simulink model "oppg5_5_e"  (R2015a)
settings: Solver=ode45  StartTime=0.0  StopTime=600  RelTol=1e-3
values from neighbouring files (symbols this model uses):
  K_pd = sqrt(T_f^2*omega_c^4+omega_c^2)/K    [oppg5_3_a.m]
  T = double(T)    [FindParam.m]    (also in oppg5_3_a.m)
  T_f = -1/(omega_c*tan(130*pi/180))    [oppg5_3_a.m]
libraries: simulink x2
settings Model: Creator=markh  LastModifiedBy=mikhailv
settings DataIOCC: SignalLoggingSaveFormat=ModelDataLogs  SignalLoggingName=sigsOut
settings OptimizationCC: InitFltsAndDblsToZero=on
settings DebuggingCC: SaveWithParameterizedLinksMsg=none  UnderspecifiedInitializationDetection=Classic  MergeDetectMultiDrivingBlocksExec=none  SignalResolutionControl=TryResolveAllWithWarning  MultiTaskDSMMsg=warning  MultiTaskCondExecSysMsg=none  FcnCallInpInsideContextMsg=UseLocalSettings  StateNameClashWarn=warning
settings HardwareCC: TargetUnknown=on
settings GRTTargetCC: TargetFcnLib=ansi_tfl_tmw.mat  CombineOutputUpdateFcns=off  GRTInterface=on

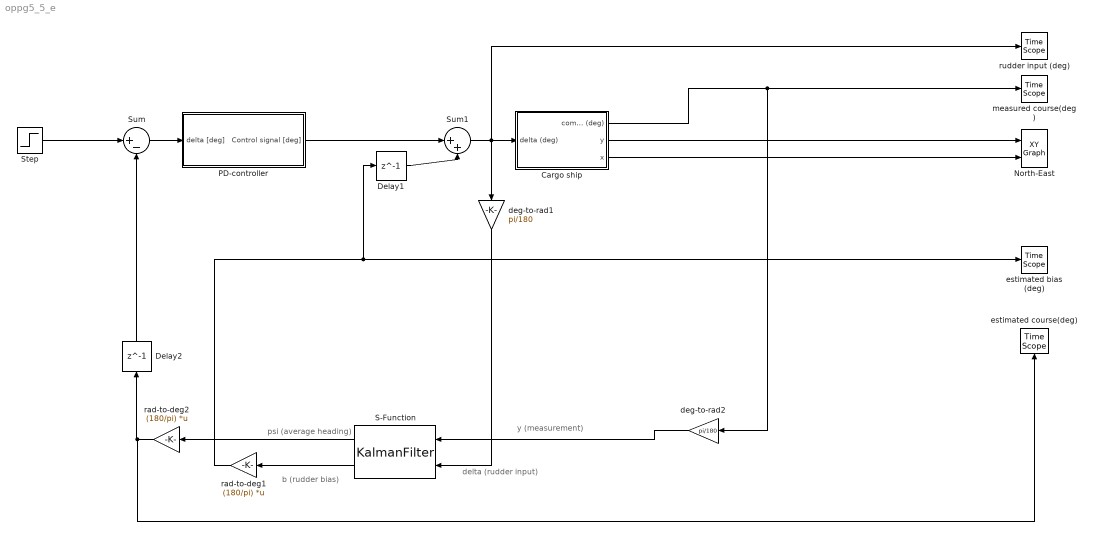
== system oppg5_5_e ==
  note: delta (rudder input)
  note: y (measurement)
  note: b (rudder bias)
  note: psi (average heading)
  Cargo ship : Subsystem  mask(Simple shipmodel for a cargo ship){noise=on, current=on, logic=on}
      mask prompts: noise "measurement noise"; logic "waves"
      mask help:
      | Measurement noise:
      | 	checked = noise on
      | 	unchecked = noise off
      |
      | Current:
      | 	checked = current on
      | 	unchecked = current off
      |
      | Waves:
      | 	checked = waves on
      | 	unchecked = waves off
      |
      | Author: Jørgen Spjøtvold, 9/10-2003
      | TTK 4115 Linear system theory.
      | Modified by Jostein Bakkeheim 26/10-2006
  Delay1 : Delay  DelayLength=1  InitialCondition=0
  Delay2 : Delay  DelayLength=1  InitialCondition=0
  North-East : simulink/Sinks/XY Graph  xmin=-5000  xmax=5000  ymin=-5000  ymax=5000  st=-1
  PD-controller : Subsystem
  S-Function : S-Function  FunctionName=KalmanFilter
  Step : Step  After=30  SampleTime=0
  Sum : Sum  Inputs=|+-  AccumDataTypeStr=double  OutDataTypeStr=double  InputSameDT=on  LockScale=on
  Sum1 : Sum  Inputs=|++  AccumDataTypeStr=double  OutDataTypeStr=double  InputSameDT=on  LockScale=on
  deg-to-rad1 : Gain  Gain=pi/180
  deg-to-rad2 : Gain  Gain=pi/180
  estimated bias (deg) : TimeScope
  estimated course(deg) : TimeScope
  measured course(deg) : TimeScope
  rad-to-deg1 : Gain  Gain=(180/pi)  Multiplication=Matrix(K*u)
  rad-to-deg2 : Gain  Gain=(180/pi)  Multiplication=Matrix(K*u)
  rudder input (deg) : TimeScope
  wires:
  Cargo ship/3(x) -> North-East/2
  Cargo ship/2(y) -> North-East/1
  Cargo ship/1(compass (deg)) -> deg-to-rad2/1, measured course(deg)/1
  Step/1 -> Sum/1
  Sum/1 -> PD-controller/1(delta [deg])
  deg-to-rad1/1 -> S-Function/2
  deg-to-rad2/1 -> S-Function/1
  rad-to-deg1/1 -> estimated bias (deg)/1, Delay1/1
  S-Function/2 -> rad-to-deg1/1
  PD-controller/1(Control signal [deg]) -> Sum1/1
  Sum1/1 -> rudder input (deg)/1, deg-to-rad1/1, Cargo ship/1(delta (deg))
  Delay1/1 -> Sum1/2
  S-Function/1 -> rad-to-deg2/1
  Delay2/1 -> Sum/2
  rad-to-deg2/1 -> estimated course(deg)/1, Delay2/1

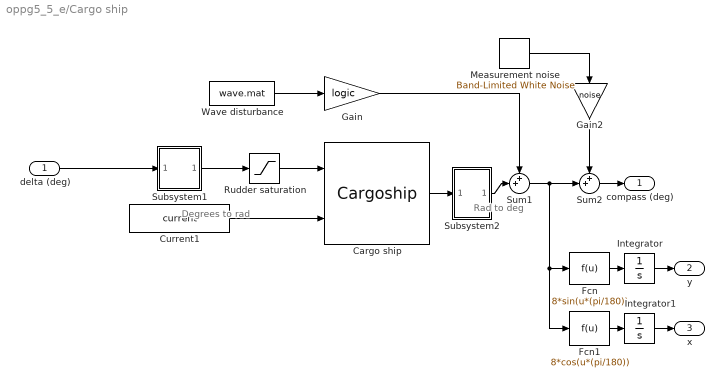
== system oppg5_5_e/Cargo ship ==
  note: Degrees to rad
  note: Rad to deg
  delta (deg) : Inport
  Cargo ship : S-Function  FunctionName=Cargoship  mask(Cargo ship){}
      mask help:
      | S-function which simulates a cargo ship.
      |
      | Author: Jørgen Spjøtvold
      | 20.10-2003
      | Modified by Jostein Bakkeheim 27.10.2006
  Current1 : Constant  Value=current
  Fcn : Fcn  Expr=8*sin(u*(pi/180))
  Fcn1 : Fcn  Expr=8*cos(u*(pi/180))
  Gain : Gain  Gain=logic  SaturateOnIntegerOverflow=on  OutDataTypeStr=Inherit: Same as input  ParamDataTypeStr=Inherit: Same as input
  Gain2 : Gain  Gain=noise  SaturateOnIntegerOverflow=on  OutDataTypeStr=Inherit: Same as input  ParamDataTypeStr=Inherit: Same as input
  Integrator : Integrator
  Integrator1 : Integrator
  Measurement noise : simulink/Sources/Band-Limited White Noise  Cov=[0.001]  Ts=.5  seed=[23341]
  Rudder saturation : Saturate  UpperLimit=45*(pi/180)  LowerLimit=-45*(pi/180)
  Subsystem1 : Subsystem  mask(degrees to radians){}
      mask help: Converts degrees to radians
      mask Display: fprintf('D2R');
  Subsystem2 : Subsystem  mask(radians to degrees){}
      mask help: Converts radians to degrees
      mask Display: fprintf('R2D');
  Sum1 : Sum  Inputs=++|  SaturateOnIntegerOverflow=on
  Sum2 : Sum  Inputs=++|  SaturateOnIntegerOverflow=on
  Wave disturbance : FromFile  FileName=wave.mat  SampleTime=0
  compass (deg) : Outport
  y : Outport  Port=2
  x : Outport  Port=3
  wires:
  delta (deg)/1 -> Subsystem1/1(In1)
  Fcn/1 -> Integrator/1
  Integrator/1 -> y/1
  Fcn1/1 -> Integrator1/1
  Integrator1/1 -> x/1
  Wave disturbance/1 -> Gain/1
  Subsystem2/1(Out1) -> Sum1/2
  Gain/1 -> Sum1/1
  Sum1/1 -> Fcn/1, Fcn1/1, Sum2/2
  Cargo ship/1 -> Subsystem2/1(In1)
  Subsystem1/1(Out1) -> Rudder saturation/1
  Rudder saturation/1 -> Cargo ship/1
  Sum2/1 -> compass (deg)/1
  Measurement noise/1 -> Gain2/1
  Gain2/1 -> Sum2/1
  Current1/1 -> Cargo ship/2

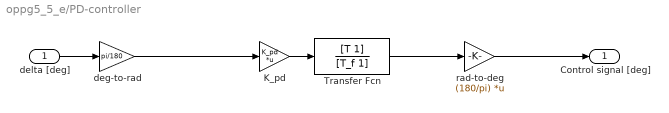
== system oppg5_5_e/PD-controller ==
  delta [deg] : Inport
  K_pd : Gain  Gain=K_pd  Multiplication=Matrix(K*u)
  Transfer Fcn : TransferFcn  Numerator=[T 1]  Denominator=[T_f 1]
  deg-to-rad : Gain  Gain=pi/180
  rad-to-deg : Gain  Gain=(180/pi)  Multiplication=Matrix(K*u)
  Control signal [deg] : Outport
  wires:
  delta [deg]/1 -> deg-to-rad/1
  Transfer Fcn/1 -> rad-to-deg/1
  rad-to-deg/1 -> Control signal [deg]/1
  K_pd/1 -> Transfer Fcn/1
  deg-to-rad/1 -> K_pd/1

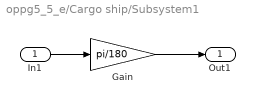
== system oppg5_5_e/Cargo ship/Subsystem1 ==
  In1 : Inport
  Gain : Gain  Gain=pi/180  SaturateOnIntegerOverflow=on  OutDataTypeStr=Inherit: Same as input  ParamDataTypeStr=Inherit: Same as input
  Out1 : Outport
  wires:
  Gain/1 -> Out1/1
  In1/1 -> Gain/1

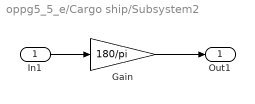
== system oppg5_5_e/Cargo ship/Subsystem2 ==
  In1 : Inport
  Gain : Gain  Gain=180/pi  SaturateOnIntegerOverflow=on  OutDataTypeStr=Inherit: Same as input  ParamDataTypeStr=Inherit: Same as input
  Out1 : Outport
  wires:
  Gain/1 -> Out1/1
  In1/1 -> Gain/1
